simulink model "hyd_hyb_2_int_cont_Final"  (Simulink 8.2)
settings: Solver=ode4  StartTime=0  StopTime=3005  FixedStep=0.01  MaxStep=.4  RelTol=1e-8
InitFcn:
  | const_3_new
values from neighbouring files (symbols this model uses):
  Af = 6.3    [brk_enrg.m]    (also in brk_enrg_1.m)
  BSFC_906_205 = [3.5684 4.3466 5.1668 6.0769 6.988 7.8992 8.8104 9.7336 10.8548 11.9809 13.1112 14.2571 ... (663 elements, 39x17)]    [BSFC_map_906_205.mat]
  Cd = 0.55    [brk_enrg.m]    (also in brk_enrg_1.m)
  den = 1.202    [brk_enrg.m]    (also in brk_enrg_1.m)
  fr = 0.01    [brk_enrg.m]    (also in brk_enrg_1.m)
undefined symbols (not defined in the file or in its folder): clutchRise, down_spd_2, down_spd_3, down_spd_4, down_spd_c, Driving_Cycle, fuel_density, gearshift, I_wheel, Idle_spd_eng_906, M1_hydr, p_v_15, pmax_125, qv_125, Rw, sec_eng_sfc_map, T0, T1, T_max_906, T_min, TC_spd_ratio_max, teta_new_10, torque_convertor, Twait, up_spd_1, up_spd_2, up_spd_3, up_spd_c, v_p_10, v_p_15, v_p_5
libraries: neural x1742, fl_lib x43, nesl_utility x30, sdl_lib x14, simulink x4, simulink_need_slupdate x1
(part 8 of 26)

== system hyd_hyb_2_int_cont_Final/controller1/optimized controller/SOC under 0.5/col_c_d1/net_col_c_d_4_5/Layer 2/LW{2,1} ==
  "ad{2,1}" : Inport  PortDimensions=30
  "IW{2,1}(1,:)'" : Constant  Value=[0.31275731661233508;-0.26985087230257487;0.14779831350765515;0.19073627614307115;0.17869846468081163;-0.4076498321664353;-0.12320323028555259;0.5405778511547239;0.12006388689999251;0.18148367011505864;0.31300573312230928;-0.24996102840664408;-0.26441353396742651;-0.31321873567065162;0.11622017278684436;-0.51269043087096478;0.24925186624599799;-0.51621146910877935;0.33750880398751393;-0.047875273652552772;0.054833649657576623;0.26144850973430128;0.31026665108346058;-0.1108382642077653;-0.23081134064217226;-0.35278496429078965;-0.10237565125670281;-0.21516087744082762;-0.48197610020281068;-0.1586790161425666]
  "IW{2,1}(10,:)'" : Constant  Value=[0.45438550635207459;-0.077905563294043856;0.064273027441706682;0.077966478501816538;0.10808472120474266;0.10911467704478268;-0.16023482762816665;0.18940926466521521;-0.21540812220195904;-0.44805812339676698;0.2672054384669737;-0.26792651540227419;0.20075923623002886;-0.22761094433996942;-0.095380404158750848;-0.084613269916532077;-0.13414255984912157;0.017595198819076098;-0.48675868307727649;0.22485563092185853;0.35538320042057187;0.041419533499156391;0.46339043665268181;0.49721579071234889;0.42207463701328973;-0.18391957358226949;0.24202005592977807;0.47408413991594811;0.52126261687656894;0.11222181265673713]
  "IW{2,1}(11,:)'" : Constant  Value=[0.39457343239192849;0.42458140946112827;-0.27287414777894187;0.067462724870659033;-0.03068429305744165;-0.11770402358430208;-0.37507142879373412;0.34598661664159674;-0.16206818607070139;-0.21370347889050573;0.39446895861921455;-0.14266125325467557;-0.14618395230039505;0.070452872197452027;0.066864440914504428;0.12451211897450633;0.012356818647122547;0.20793588176160319;0.11581661701219066;-0.35814546578829082;0.22455949634467293;0.5468167979497347;-0.55309677720618045;0.18067877568756779;0.00079594352242104113;-0.22857690375549169;-0.53472450281376172;-0.20073202836744419;-0.49233912412032937;0.40992076701468799]
  "IW{2,1}(12,:)'" : Constant  Value=[0.41350579326766701;0.21762640096045338;-0.3097139754237494;-0.2329698564124216;-0.40175947951283236;-0.23814602984300204;-0.51438263530747763;-0.20638550086744714;-0.13770761946706397;0.20930534945632584;0.46082097929918853;0.21897176978274985;-0.27255663625198434;-0.15054029720111464;-0.31656190468089873;0.33873660377538872;-0.018063524886034854;-0.36802746829566002;-0.18497782466494439;-0.19667489988898551;0.15281990588690275;0.27364171079455202;0.33039364278843469;-0.26666673631028642;-0.24425693716621172;0.040179265190829531;0.47861972776555706;0.26460968321609213;0.11706213520914137;-0.31923071600415104]
  "IW{2,1}(13,:)'" : Constant  Value=[-0.38983329555488072;0.10298134054478783;0.21048069589522062;-0.30818809919317486;0.16735156940050316;0.41375380311198673;-0.38987145223320535;-0.35565431169396255;0.22351610936772529;0.25879777713949231;-0.14184756994632572;0.43424468556067913;0.013375203965787376;-0.46400352956380603;-0.27636068442283446;-0.11336907725358317;0.08727021308118893;-0.24264501449480502;0.20756145821823418;0.27346740399021308;-0.42540340708638469;0.19736043169833001;0.44350595567853268;0.19321888665059592;0.37137571007612136;0.34439432357764344;0.27178309423110542;0.39923266521435319;0.13146686845982195;-0.11037819911004416]
  "IW{2,1}(14,:)'" : Constant  Value=[0.21882975012069514;0.1102379619120018;-0.10070141925502289;0.32743984138257093;0.51118972234674531;0.43573443039915827;-0.34375367534563284;0.28860869899214936;-0.027302686712575221;-0.33514454875747118;-0.42624595937362442;0.33248754422370219;-0.21807042688745035;-0.52802984846735068;0.18057289640456653;0.38725540109825934;0.29859268669837774;0.11535303256146118;0.31188442053164722;-0.15890248352815453;-0.061821527024561958;0.11984764110158726;-0.036239661265500982;0.42448419345038174;-0.0040841624827879621;-0.35047521428981115;0.36539965174890987;-0.25151482552180904;0.0043691747446089387;-0.14143232802150388]
  "IW{2,1}(15,:)'" : Constant  Value=[0.40647338431822938;-0.20001708935167542;-0.51281094464128818;0.049782981157163765;-0.17920999529625167;-0.27329699265418117;0.26962913809040551;0.47716366967560603;0.53696090038913025;-0.31255154459434042;-0.029745540476640381;0.1866160633838472;-0.33905178678588266;0.29106755325766553;-0.25821542422978266;-0.24029339121230353;-0.0035892080936714759;0.3194228020317908;0.33761714149176425;0.22697923201352907;-0.077978749273528103;0.050585502149808108;-0.22800546330759139;-0.45058281599612149;0.31595194999031218;0.44829307353340181;-0.27877965028572105;-0.21315229504655123;0.21126039289530585;0.32371351590829367]
  "IW{2,1}(16,:)'" : Constant  Value=[0.068233289188800172;-0.35511628123062366;-0.13456127181794694;-0.11816939495311189;0.35215637018833529;-0.41653092957567556;0.27862712938625833;0.11914056411175804;0.35499529655056261;-0.10061969322539223;0.14120075828841808;0.39501967548068662;0.22237098694536198;0.22753039224917407;-0.1912161648101082;-0.053532058431284404;0.43330060830843981;-0.40135538410096994;0.12027399398626523;-0.29127748746366555;0.22073000400657264;-0.52488192987064708;0.04552877510689797;0.032071827906611852;0.25221796966568777;-0.1246298134168777;0.48349959007046628;0.35217749374902163;-0.43579154396212266;-0.34095381824640847]
  "IW{2,1}(17,:)'" : Constant  Value=[-0.24102258277888214;0.42237910973632548;0.3732244626117559;0.2645155665316376;0.063016448033312911;-0.078422893492473861;0.302057424776629;0.35972686797948694;-0.41651868843111522;0.49899190855904718;-0.46472265979404825;0.005949808915848195;-0.41033968769219381;0.12309139438986795;-0.072517893553310162;0.43612188032541083;-0.336647838886863;0.39085946595790944;-0.32212246749708662;0.014697880621202938;0.12960680979224209;0.10392912461439244;0.074160942133394012;-0.46779281255777821;0.20515478936828335;0.25081088087070574;-0.10698219453587313;-0.21295991077406673;-0.21297824442243884;0.21837942947106137]
  "IW{2,1}(18,:)'" : Constant  Value=[0.059759050225267778;-0.27791706807936212;-0.35008479273333992;0.24878321748016538;0.075872716130115328;-0.0676945295150779;-0.44124907434319061;0.35000632127664316;0.38533241526586348;-0.12361078789315258;-0.082779322297490271;0.15999329415881977;0.042356342806022261;0.29030424704665431;-0.51698206134190861;0.21320259619178908;0.4121019278486926;0.37465473694615287;-0.25132108070492681;-0.11007359828242552;-0.33015522076856618;0.18798249136039627;0.18204609562084603;-0.39665944445609236;-0.41154660905580748;-0.16994986605823159;-0.1692955872746989;-0.084005493488811103;-0.47131807612986337;-0.45578642456255264]
  "IW{2,1}(19,:)'" : Constant  Value=[-0.47886938227031417;0.032469457537400305;-0.25542104742245059;-0.26167394587019804;-0.10238940058752172;0.09748971581301949;0.10986467030249047;-0.22034914411988779;0.26410419478307628;0.19984648446248054;0.10272919448576125;-0.56053811290237565;0.25628511943482707;-0.16813290569704722;0.39759444526884469;0.56965220071070788;0.38494247411175653;0.16530272179566097;-0.048376693521673432;0.21177807584289449;0.37575026242104831;0.30453417835192959;0.31565094074247002;0.1676691940210048;-0.033954839293835484;-0.28130350691137318;0.18751282661063398;0.29791372323587106;0.48208294523816858;-0.24731324303734542]
  "IW{2,1}(2,:)'" : Constant  Value=[0.16485594905702061;0.41958460563899208;-0.087556982214553172;0.099659077192037468;-0.34322740388705358;-0.3233151486552453;-0.41887378222277061;0.046432114993733058;-0.04898360854476292;0.16153529016460713;0.28844117833541272;-0.29776282115080782;0.25010799495268621;-0.50504804649059543;0.23860604320730203;-0.34818567250330251;0.33046575769726333;-0.46398401002715511;0.09588243880572192;-0.28059551643412539;-0.25844161306811819;0.19187556916319429;-0.22646588144013996;-0.12620457794262144;-0.38984869350840334;0.50675143299656611;0.11659348313501641;0.11930517585189776;-0.38665943551255716;0.15213966711994284]
  "IW{2,1}(20,:)'" : Constant  Value=[-0.50349152720019708;-0.15010554830208991;0.04823860371701947;0.21563733179354533;0.17870399256241923;0.36223693131943974;-0.17259449670673224;-0.15585032550862551;-0.30294761986714053;0.40528052511574736;0.062050664964907888;-0.029356423222545683;-0.29477014410269187;0.058391152070021719;-0.47589128512679713;0.53116788114847968;0.1868250849425496;0.040929221667824277;0.38990550796746748;0.24300137252896023;0.10615772766965213;-0.12223235512275682;-0.38620447778361577;0.10284616000000632;-0.53191757250801641;0.060123296195749305;0.42009066845053133;-0.081139615013162442;0.28050737924076169;-0.39610717394304934]
  "IW{2,1}(21,:)'" : Constant  Value=[0.27654849170357604;0.44000998144944226;0.34978032343014748;0.16287626128560476;-0.31106448364869971;0.2712986975363621;0.17477184643602001;-0.040994417241635855;0.040756820710299513;-0.32217945823032945;0.033526998625739449;0.28083486484077141;0.07527788850813795;0.031141752002320815;-0.13842179269689114;-0.44467088615542294;0.16343581497338305;-0.25175895155410183;0.37296608238294682;-0.26225689114314404;0.036532039732935541;0.57172449283776772;0.11563544110226888;-0.41021444626899761;0.24900514830006129;0.29631891929786808;0.42548416020169089;0.42501941439136554;0.66763009748879998;0.03027871495198993]
  "IW{2,1}(22,:)'" : Constant  Value=[0.38175362027160537;-0.2376980384911867;-0.30063107682478601;-0.33881306444168069;0.17849746917857029;-0.34964626211640071;0.47826477896920283;-0.45640710628278391;-0.27942561203021932;0.40006277245588362;0.12139177090538589;0.23428665944684432;0.47448510322777709;0.0048315672861399079;-0.062689816480599722;0.060400310154686547;-0.20714240476303258;-0.42676738802132902;0.33105522009343091;0.063936510689872036;-0.17953036149592752;-0.27004097229269541;0.45556337239058609;-0.18429429231486444;-0.34003366383251599;0.24510978349593487;-0.1936015912949566;-0.21466624872492407;0.14985155313151818;0.054107134676608881]
  "IW{2,1}(23,:)'" : Constant  Value=[0.19208517656566945;-0.23756553933116847;-0.40298748221062619;0.315881501215938;0.33300767958814698;0.054607137245660312;0.070510839064599679;0.25843945839112381;-0.47818192403809279;-0.22121986735846599;-0.42796937877860231;0.28019957286856068;-0.42271140569854398;0.24074409826905843;-0.2382457659414558;0.31288621521010146;-0.10634533622057268;-0.42795872100881838;0.33242045568973272;0.27235300570836396;0.4452188850608414;0.25216641636573384;0.42859453638665451;0.042237698775830494;-0.010407092153751055;0.27847694370500309;0.037030252368509826;0.24700161997172382;-0.2740168070269105;-0.051812001981064143]
  "IW{2,1}(24,:)'" : Constant  Value=[-0.25041942582150839;-0.4783743097785057;0.33758877202355092;-0.35771582757284054;-0.069784976792996542;-0.18183718522479581;-0.29647307869149248;-0.01258022132651891;-0.38608590463206277;-0.17128957156155242;0.28378323654610887;-0.1232662979796499;-0.034840090696733474;-0.21583788403895016;-0.35856711536397545;0.27291622414266103;-0.48944471164387804;-0.17030385013592783;-0.31970851699994202;0.17182723354569193;-0.050945541622091077;-0.2331708593756367;-0.0011402081132685206;0.40596696938193017;0.30363557399044233;-0.2771351555329063;0.35320261019636923;-0.27312545966154628;0.50923636237666603;0.22586347700180542]
  "IW{2,1}(25,:)'" : Constant  Value=[0.32349444512379921;0.074648383376890656;0.18340658341772714;0.43907131187832443;0.24465430553770609;0.23034266690144972;0.47224773188761382;-0.039851790753156688;-0.28799592424079162;0.46792175397215163;-0.052747978840832654;0.18850645864976925;-0.23554460115113637;-0.19364311776843482;0.35316221950874893;0.44064660342413975;0.18917215303582707;-0.12420884828585119;0.40538631794931379;0.22819341411136568;0.059594500015362512;0.28343720639866427;-0.45140839586712117;0.1478703357973816;0.30076697778334688;0.15221057482232195;0.035957199643899887;-0.17933932303548003;-0.41443602301923138;0.42878258387315454]
  "IW{2,1}(26,:)'" : Constant  Value=[0.36591493875311448;0.42528293161766884;-0.30435369071635565;0.14276477985755814;-0.04495075026453995;0.19809379202781327;0.51087121120446755;0.21486333322079815;-0.34059850815575499;0.084745163469986964;-0.30926516084598771;-0.07546102676902644;-0.12460229619037608;0.18508313015789429;0.12897811993832092;-0.22442795556708969;0.019023619473468013;0.34747781394647176;-0.37296250313818691;-0.028844860117835443;0.30287166816632488;-0.18991160260759973;-0.41896864492380009;0.0032567424690979675;-0.28457586214599073;0.21844863504622525;0.18315065831218991;-0.46689768004420179;0.65930160457142706;-0.50391368734202047]
  "IW{2,1}(27,:)'" : Constant  Value=[-0.45165726459295841;0.18685298448002466;-0.0090335448745681585;-0.52954877861384042;-0.14477143023223485;0.045597100123252285;-0.29536340634700303;-0.19327933685493373;0.24862380838491852;0.19703321893290365;0.5107467939404432;-0.16533346090025589;-0.26226009715655274;-0.15632117807422943;-0.063571615898426373;0.55995701861756586;-0.53001173127896606;-0.19441677800206064;0.076824338048925925;-0.11179108588524951;-0.14135238157903199;0.39349867681877754;0.023404631751319238;0.37216463490856705;0.53159287863188354;-0.282683317094924;-0.1273085783656768;-0.11809939138651696;0.062648977706862341;0.01948150734503756]
  "IW{2,1}(28,:)'" : Constant  Value=[-0.58060952775684338;-0.22557606247832096;0.52097869943267794;-0.19586163071942558;0.0062674764494588262;-0.066850020962621756;0.20177734453309737;-0.27847284591627308;0.33847362494561467;0.35269036115819041;0.39821372354421114;-0.075296913241820349;-0.2104646699645738;0.44653380119651459;-0.18745831379084438;-0.60540044413148164;-0.082560268753580454;0.010533100539155408;0.093177597410024335;0.029253479090595141;-0.035674987634033255;-0.20045674250673423;-0.30562918019644403;-0.24631105348707522;0.045490458801701883;0.059752260576021003;0.55791046780256159;0.19353601707602536;0.28902863117259614;0.066799928097732178]
  "IW{2,1}(29,:)'" : Constant  Value=[0.200626701170141;0.11341200725191816;0.25400945898747868;-0.29711962816610615;-0.25863315355850092;0.35744982028032246;-0.5080920038212503;0.58181325676261442;-0.097398879041334083;-0.12638833145718376;-0.10014932495998892;-0.28239825293861465;-0.2339851544517525;0.14485834314410745;-0.25498351212539166;0.045186437575171177;0.59327181045491273;-0.60524360933909438;0.25456298981177006;-0.18584367266637661;0.12303436253633954;-0.042955730385764286;0.42151102793510242;-0.23533227271142015;0.10481495152121964;0.0024264444668975877;-0.032072789036909792;0.28820697053753419;-0.24353411968483479;0.17434993503616078]
  "IW{2,1}(3,:)'" : Constant  Value=[0.3459096676297157;-0.11796751712458815;0.46227598264851438;0.14263353014580396;0.34214145196121382;0.067536028640059004;-0.4308090682770192;-0.26595770030532756;-0.40464381327048471;-0.41297978470556329;-0.083143061155957307;-0.2213102003231478;0.28674899904423712;-0.25566004614728211;-0.2637262681895613;-0.19672965570919757;0.42630776831842748;-0.23603035795505956;0.18479113555339288;0.13330554053305646;-0.44289673634078358;-0.22028406519497015;-0.071392960615195372;-0.2619638898003428;-0.27848765975481171;0.31573980431370213;-0.29837469379576242;-0.4458157730139885;0.064506187512735597;-0.11504288424397838]
  "IW{2,1}(30,:)'" : Constant  Value=[0.15190325397518098;-0.34216215066573985;-0.39814751560646894;-0.42943267994355339;-0.21875047919699234;-0.21287914075563277;-0.27073826951352659;-0.42295417300718602;0.32460992703246305;-0.43774963439841746;0.061558139773068475;-0.019684675811075684;0.42020559123125811;-0.39776452768660175;-0.5234335532592449;-0.16168817301124472;0.14003142322982184;0.10628363934677905;-0.086823016807298495;-0.046194531903006285;-0.033725503218865346;-0.41006731661327178;-0.34684589361002549;0.082045516770265753;-0.28831677388251697;0.38628769766659182;0.28636646919507447;-0.14510905709409513;0.29510810475862387;-0.21942176632829943]
  "IW{2,1}(31,:)'" : Constant  Value=[-0.39196147587405461;-0.30484384520281688;0.32339020886236586;-0.24533783720737751;-0.28243060314126101;0.35853256400686745;-0.096180248562639889;-0.3031052656978025;-0.46296078164800541;0.017110740095564039;0.24319533946695593;-0.14594960536939233;-0.46901714224314928;-0.42991556788729024;-0.24347837627827257;0.49572366809363572;-0.3711206454426727;-0.078473534413682378;-0.18768615924301743;-0.19917658263020099;-0.36562820167011711;-0.060476596214022328;0.22652353361504782;0.082677122740594522;-0.27809312170130696;0.14116400393821171;-0.37520933679946206;0.20713872373871514;-0.12846495534626934;-0.26230599104356522]
  "IW{2,1}(32,:)'" : Constant  Value=[-0.27915563919657271;0.0031543366869891116;-0.074356213945820829;0.60541914834384591;0.21906474630133854;0.053542864961575495;-0.41393610408740883;0.049831763478782272;-0.59172997102716274;-0.21372816909418876;-0.47611585362483089;0.024910784918673722;-0.6694666312496329;0.082460309831931727;-0.17015304403916198;-0.070164320290546353;0.047563633318013374;-0.34828596499173975;0.039615165090038554;-0.22770922258295684;0.12685346317662261;0.5812308928526484;-0.26687408138421853;-0.10678767449453988;-0.30871960935658288;0.080909724361547933;-0.065676115606442972;-0.17599364507922607;-0.15345393026672444;-0.13957577397509063]
  "IW{2,1}(33,:)'" : Constant  Value=[-0.14241530488200782;-0.42802886140837171;0.22382159633187695;-0.23395685062514587;-0.43289738365933766;-0.33881337748403562;-0.2807740627158769;-0.18296096952563212;0.33633354136552684;-0.095685317058735384;-0.36551851743406943;0.45398299496209066;-0.14601089686704719;0.39142342911155814;-0.27831665329158656;0.21541539538043869;-0.36029628835130523;-0.43108890247934833;0.18302081726576166;0.084393873101736697;0.3259336830432813;0.41589742614527048;0.26087955589125039;-0.21282332443442339;-0.24557835715225795;-0.027545930655320287;-0.31727289221876193;-0.26420356879217649;0.15847775495593014;0.18198182070612359]
  "IW{2,1}(34,:)'" : Constant  Value=[-0.1080813176840188;0.031877423816805729;0.43003917155021437;-0.19446938568529362;-0.4638454953879948;-0.23757477543062727;0.032996428279117494;-0.23966793739279438;0.38410933344413728;0.15240169782027815;-0.42872348965582635;-0.020835572776745432;0.17700773516150659;0.48990883523550122;0.37097995759145441;-0.30512589395578371;-0.44608773131815127;0.32579486658577667;0.39636767324860256;0.1807027895135021;0.23749883582488848;-0.24971507549780828;-0.36185798007397568;0.48185320598392634;-0.11417150403539712;-0.072485959616476234;-0.18977680507334568;0.0087344840836283879;0.19591929810703587;-0.1611155049720481]
  "IW{2,1}(35,:)'" : Constant  Value=[0.28637756011481041;-0.01883311693596772;0.4032250294391555;-0.1620436547326822;-0.51840640598156196;-0.43210195154936415;0.29892194265780975;-0.010068380822181065;-0.032801409050717385;-0.094579120494082611;0.084606294379177452;-0.3250088029757065;-0.17473214707481291;-0.21568918324783523;-0.43287752741456603;0.46279201783067719;-0.002324495961844919;0.13076008214567994;-0.28600464486555599;-0.23721237794517117;0.11391355774762742;-0.41839662000656508;-0.51413807719874494;0.18575832928932814;0.18961472877535523;-0.089024071548704786;0.48390714533162726;0.11636984161140511;0.34653536649007477;-0.17927531322005694]
  "IW{2,1}(36,:)'" : Constant  Value=[-0.36210314109763053;0.14584188290398084;-0.35438442449050594;0.32315450009904317;0.18434784726834644;0.38493084551990348;-0.096535485247892447;-0.18658324859701786;-0.046754406456686326;0.51074777088191625;0.31481372129285495;0.37681683213926354;-0.32036486099036615;0.017548820888744331;0.4009661821533998;0.098167186415540009;0.23451840361056001;0.39521897549836915;0.041940753905107306;0.28840714311974119;0.092321041979203114;0.25009242632983703;0.25803285198791565;-0.46282207162139155;0.40890961979162882;0.021747727427568642;-0.49511963345440418;-0.20447453933880586;0.047925656474884122;0.14473490628736754]
  "IW{2,1}(37,:)'" : Constant  Value=[0.30895980101971848;0.2205995057081224;0.014215062392222162;-0.35743246531383871;0.078114912171393075;-0.3716774172840871;0.18963429706101939;0.094014671548542858;-0.30483996969855698;0.27231359653796966;-0.21558939931622154;0.20737577142209412;-0.33794212840815074;-0.16422042277311097;-0.432186262416135;0.44347392277162362;-0.28376178074835973;0.092808417192934811;0.23982683239387254;-0.057619954301717249;-0.1502789954807599;-0.50024378241445777;-0.055461327531646114;0.15889498771577498;-0.49528223882524575;0.54437730654311189;-0.33165473512905069;-0.26995389111620571;0.20230457029389584;0.083413067871219063]
  "IW{2,1}(38,:)'" : Constant  Value=[0.31376155073349921;0.38735585542746392;0.11982352708142101;-0.44485010346037318;0.2538529549617653;0.12326898087066515;0.19627230873225621;-0.12292507361069381;0.44732019656864452;0.21381392787092793;-0.10540473725430266;0.046547911838308614;-0.26005530486766804;-0.092360969592290634;-0.35643113638449714;-0.30793831072341116;0.42038732950729013;0.40916985478650209;0.22768604915972937;-0.34754216788287967;-0.098971341532745671;0.39545233206496044;-0.41400939765243283;-0.1522799472065576;0.16999513541993228;-0.30420322783241793;0.094578321305834573;-0.26622295727616196;0.36998948162013501;0.37491396323200438]
  "IW{2,1}(39,:)'" : Constant  Value=[-0.0020064593389496049;0.42463890271185478;-0.084869246006223503;0.13312921673087996;-0.35561987529069944;-0.1631643953339536;-0.10922694340892829;-0.06765434448875729;0.037078984117479584;0.039871739277738717;-0.14593915974365232;0.43656333330665248;0.26261588008845604;-0.39756482931894077;-0.41914777810315396;-0.41721262966073996;0.49922918699183166;0.097945865589809181;-0.25934109090236468;-0.40641397794973788;-0.49046253407477991;0.23959196411459993;0.022923979689467112;0.26567613392988421;0.34004535213417464;-0.48963607367670614;0.17405455279805812;-0.11888857301090927;-0.29101122979555866;0.022759802472809038]
  "IW{2,1}(4,:)'" : Constant  Value=[0.24884602764519553;0.011662817403598679;0.30004204405401175;-0.30213030285491976;-0.37240048328027758;-0.063612854437861036;0.16885727465472147;-0.19920232018388431;-0.4327371635069609;0.3281653159173003;0.24440163725476829;-0.40961038191572063;-0.32071974797282893;-0.22574883055005474;-0.40258802248002623;-0.38044163556309479;0.28940501837107774;-0.36724248494394268;-0.36539679359632593;-0.13576889895403829;0.096013382386674506;0.15767164369658879;-0.35887994422675973;-0.26090216467487937;-0.35986426731161514;-0.44831164855973205;0.19102962307798715;0.12934044546397921;-0.090685632702068183;0.24438127240792426]
  "IW{2,1}(40,:)'" : Constant  Value=[0.47231305767361814;-0.4435329241076687;-0.29471890313503751;-0.29445184768907751;-0.1288902727338922;0.42178628341168645;-0.17367845551935812;-0.011520243983458654;0.063013213396622705;-0.30807790612722352;-0.10467980927399435;-0.34730373262865949;0.032801004445701464;0.0012963986235965555;-0.13888340651489126;0.32696783648073474;-0.31576075422582089;0.21365430733274085;-0.4134871672491357;0.31745202000616701;-0.12498690934146456;-0.2947331210328587;0.45129695059181368;0.43023017404594532;-0.35936441760492538;-0.44554958440007569;0.17420016060189544;0.12202951393332437;0.20479294535271642;-0.077817926858881906]
  "IW{2,1}(5,:)'" : Constant  Value=[-0.062901709304139783;0.32341137965665484;0.050527689980782754;-0.16487151299127989;-0.045815962388067497;0.50511421457259975;-0.18013089336815724;0.061715070505560118;0.28235840385390576;-0.39856132729554111;0.0023061732376174794;-0.23449982892962193;0.38952129699583593;-0.011440048982628416;0.40942338391488875;-0.39827020000003011;0.023525814677469354;-0.2186305674801248;0.52230031676125732;0.41492987436367007;-0.42941454695237141;-0.15360167182139192;0.27769917090917323;-0.4266750314682079;0.35265544711904667;-0.048369340187480195;0.045767014999578512;-0.019588517841915076;-0.36491651405831882;0.30534704709780569]
  "IW{2,1}(6,:)'" : Constant  Value=[0.14649388353113663;-0.22457556384651209;0.41114328992622839;-0.40380519063788617;0.46424038683218355;-0.34306115074364552;-0.40919766016808684;-0.048929718916915249;-0.41471276760485898;-0.28448059873982734;0.42312029090984776;-0.10463115287581726;-0.13722175612637078;0.11679976409816603;-0.22948999051804081;0.064769205503860949;-0.24089725871610537;-0.23693643690607052;-0.29211385277033741;0.073667883044920585;-0.46627822849915135;-0.25574129709186616;-0.103535859979867;-0.2874562200965296;-0.27565493511549399;-0.20832958498408963;0.47443704695435779;0.36303048561885215;0.14695330736401896;0.046696723471653406]
  "IW{2,1}(7,:)'" : Constant  Value=[-0.28369330135027643;-0.28247025426586919;-0.29327005551695901;0.33716826498283092;0.27667110389940391;-0.10852914106983955;-0.39616325954735659;0.31312232949019919;0.16069907041519635;-0.21407336364033694;0.29314107740163425;-0.082119025675407215;0.27377487239493759;0.010940682067417256;0.198272649173522;0.40906242406446958;-0.15188119293446137;-0.35309753913457093;-0.38016952468941689;0.40029450234037023;0.12759173703826107;-0.33040256725861405;-0.2703842078354089;0.33484452581795426;-0.35398015747574452;-0.010795853196711971;0.34312537372447;-0.053240154935927826;0.34412665912292595;0.37251434655521104]
  "IW{2,1}(8,:)'" : Constant  Value=[-0.20923284873373496;0.24554235823081641;0.27407254142511789;-0.08214097632887632;-0.21240424957991907;-0.32026505432150049;0.4388254076141479;-5.1044985481562587e-005;-0.39064340534512793;-0.4149544427086127;-0.39537804980330282;-0.34694923824881235;0.19431640822985691;-0.36321375493294389;0.14098683810873255;0.34412516279956412;-0.023064918854102036;0.20078487216987131;-0.18711800366799441;-0.29535806023912431;0.068030782603948875;-0.265067842092996;-0.12145593370504683;-0.47512489122608942;0.38230144593675691;-0.075320862525029911;-0.33328505959559945;0.39182886243929138;-0.22974155825193956;-0.44096692163984375]
  "IW{2,1}(9,:)'" : Constant  Value=[-0.38273875807747837;-0.53038263554913556;0.07663390557537525;0.3517524726482894;-0.36880503061111952;0.26994520408226053;0.1154625386840097;0.042636040009437715;0.44297428848937392;-0.38061478854327563;-0.47190766217819219;0.25615755069572643;0.3584017357215783;0.067414172681270007;-0.20091641281789024;0.213782292714123;0.077085749553810076;-0.1050348327444577;-0.28870725365274741;0.0038040324511218154;0.136175748417838;-0.34565268641657898;-0.33113569859445707;0.050391119456636949;-0.32682675250849214;-0.20582404721348957;0.36911869262913682;0.070626392320243411;-0.027000597528334495;0.46817855347483345]
  Mux : Mux  Inputs=40
  dotprod{1..40} (40 alike) : neural/Weight Functions/dotprod
  "lz{2,1}" : Outport
  wires:
  Mux/1 -> "lz{2,1}"/1
  dotprod40/1 -> Mux/40
  "IW{2,1}(40,:)'"/1 -> dotprod40/1
  dotprod39/1 -> Mux/39
  "IW{2,1}(39,:)'"/1 -> dotprod39/1
  dotprod38/1 -> Mux/38
  "IW{2,1}(38,:)'"/1 -> dotprod38/1
  dotprod37/1 -> Mux/37
  "IW{2,1}(37,:)'"/1 -> dotprod37/1
  dotprod36/1 -> Mux/36
  "IW{2,1}(36,:)'"/1 -> dotprod36/1
  dotprod35/1 -> Mux/35
  "IW{2,1}(35,:)'"/1 -> dotprod35/1
  dotprod34/1 -> Mux/34
  "IW{2,1}(34,:)'"/1 -> dotprod34/1
  dotprod33/1 -> Mux/33
  "IW{2,1}(33,:)'"/1 -> dotprod33/1
  dotprod32/1 -> Mux/32
  "IW{2,1}(32,:)'"/1 -> dotprod32/1
  dotprod31/1 -> Mux/31
  "IW{2,1}(31,:)'"/1 -> dotprod31/1
  dotprod30/1 -> Mux/30
  "IW{2,1}(30,:)'"/1 -> dotprod30/1
  dotprod29/1 -> Mux/29
  "IW{2,1}(29,:)'"/1 -> dotprod29/1
  dotprod28/1 -> Mux/28
  "IW{2,1}(28,:)'"/1 -> dotprod28/1
  dotprod27/1 -> Mux/27
  "IW{2,1}(27,:)'"/1 -> dotprod27/1
  dotprod26/1 -> Mux/26
  "IW{2,1}(26,:)'"/1 -> dotprod26/1
  dotprod25/1 -> Mux/25
  "IW{2,1}(25,:)'"/1 -> dotprod25/1
  dotprod24/1 -> Mux/24
  "IW{2,1}(24,:)'"/1 -> dotprod24/1
  dotprod23/1 -> Mux/23
  "IW{2,1}(23,:)'"/1 -> dotprod23/1
  dotprod22/1 -> Mux/22
  "IW{2,1}(22,:)'"/1 -> dotprod22/1
  dotprod21/1 -> Mux/21
  "IW{2,1}(21,:)'"/1 -> dotprod21/1
  dotprod20/1 -> Mux/20
  "IW{2,1}(20,:)'"/1 -> dotprod20/1
  dotprod19/1 -> Mux/19
  "IW{2,1}(19,:)'"/1 -> dotprod19/1
  dotprod18/1 -> Mux/18
  "IW{2,1}(18,:)'"/1 -> dotprod18/1
  dotprod17/1 -> Mux/17
  "IW{2,1}(17,:)'"/1 -> dotprod17/1
  dotprod16/1 -> Mux/16
  "IW{2,1}(16,:)'"/1 -> dotprod16/1
  dotprod15/1 -> Mux/15
  "IW{2,1}(15,:)'"/1 -> dotprod15/1
  dotprod14/1 -> Mux/14
  "IW{2,1}(14,:)'"/1 -> dotprod14/1
  dotprod13/1 -> Mux/13
  "IW{2,1}(13,:)'"/1 -> dotprod13/1
  dotprod12/1 -> Mux/12
  "IW{2,1}(12,:)'"/1 -> dotprod12/1
  dotprod11/1 -> Mux/11
  "IW{2,1}(11,:)'"/1 -> dotprod11/1
  dotprod10/1 -> Mux/10
  "IW{2,1}(10,:)'"/1 -> dotprod10/1
  dotprod9/1 -> Mux/9
  "IW{2,1}(9,:)'"/1 -> dotprod9/1
  dotprod8/1 -> Mux/8
  "IW{2,1}(8,:)'"/1 -> dotprod8/1
  dotprod7/1 -> Mux/7
  "IW{2,1}(7,:)'"/1 -> dotprod7/1
  dotprod6/1 -> Mux/6
  "IW{2,1}(6,:)'"/1 -> dotprod6/1
  dotprod5/1 -> Mux/5
  "IW{2,1}(5,:)'"/1 -> dotprod5/1
  dotprod4/1 -> Mux/4
  "IW{2,1}(4,:)'"/1 -> dotprod4/1
  dotprod3/1 -> Mux/3
  "IW{2,1}(3,:)'"/1 -> dotprod3/1
  dotprod2/1 -> Mux/2
  "IW{2,1}(2,:)'"/1 -> dotprod2/1
  dotprod1/1 -> Mux/1
  "ad{2,1}"/1 -> dotprod40/2, dotprod39/2, dotprod38/2, dotprod37/2, dotprod36/2, dotprod35/2, dotprod34/2, dotprod33/2, dotprod32/2, dotprod31/2, dotprod30/2, dotprod29/2, dotprod28/2, dotprod27/2, dotprod26/2, dotprod25/2, dotprod24/2, dotprod23/2, dotprod22/2, dotprod21/2, dotprod20/2, dotprod19/2, dotprod18/2, dotprod17/2, dotprod16/2, dotprod15/2, dotprod14/2, dotprod13/2, dotprod12/2, dotprod11/2, dotprod10/2, dotprod9/2, dotprod8/2, dotprod7/2, dotprod6/2, dotprod5/2, dotprod4/2, dotprod3/2, dotprod2/2, dotprod1/2
  "IW{2,1}(1,:)'"/1 -> dotprod1/1

== system hyd_hyb_2_int_cont_Final/controller1/optimized controller/SOC under 0.5/col_c_d1/net_col_c_d_4_5/Layer 3/Delays 1 ==
  "p{3}" : Inport  PortDimensions=40
  mux : Mux  Inputs=1
  "pd{3,2}" : Outport
  wires:
  mux/1 -> "pd{3,2}"/1
  "p{3}"/1 -> mux/1

== system hyd_hyb_2_int_cont_Final/controller1/optimized controller/SOC under 0.5/col_c_d1/net_col_c_d_4_5/Layer 3/LW{3,2} ==
  "ad{3,2}" : Inport  PortDimensions=40
  "IW{3,2}(1,:)'" : Constant  Value=[-0.43141211792559142;-0.11888165414139513;-0.22701302193417633;0.14315500955996635;-0.11268052842329422;-0.66755337377971913;-0.90374763549360537;-0.76985267606758923;-0.62023649272464287;0.19138878884193214;0.99640825481026107;0.30069820196235497;-0.90113832366665458;-0.69317441551269632;1.0524663804640109;0.40315249365778993;0.8257560441646864;-0.43196133618180077;-0.62424800501186883;0.74264769849740953;0.99995606798411707;-0.13032239355778821;0.71476098102029351;0.92404578703104456;0.075939871013732146;0.94468909976236903;0.19330991737906994;0.47787649449252922;0.89436963345916265;-0.79706254287066325;-0.01014931738240097;0.58899206441818175;0.98972787944860419;-0.19553007982111831;-0.10078290415230909;-0.26312481872565424;-0.80903105213119841;0.38143504933278732;-0.098828531512075504;0.27196209686502049]
  Mux : Mux  Inputs=1
  dotprod1 : neural/Weight Functions/dotprod
  "lz{3,2}" : Outport
  wires:
  Mux/1 -> "lz{3,2}"/1
  dotprod1/1 -> Mux/1
  "ad{3,2}"/1 -> dotprod1/2
  "IW{3,2}(1,:)'"/1 -> dotprod1/1

== system hyd_hyb_2_int_cont_Final/controller1/optimized controller/SOC under 0.5/col_e_f/net_col_e_f_2_4/Layer 1/Delays 1 ==
  "p{1}" : Inport  PortDimensions=2
  mux : Mux  Inputs=1
  "pd{1,1}" : Outport
  wires:
  "p{1}"/1 -> mux/1
  mux/1 -> "pd{1,1}"/1

== system hyd_hyb_2_int_cont_Final/controller1/optimized controller/SOC under 0.5/col_e_f/net_col_e_f_2_4/Layer 1/IW{1,1} ==
  "pd{1,1}" : Inport  PortDimensions=2
  "IW{1,1}(1,:)'" : Constant  Value=[-2.6649767493760956;-1.5305742272763116]
  "IW{1,1}(2,:)'" : Constant  Value=[-2.686906454238835;-1.6060629338452583]
  "IW{1,1}(3,:)'" : Constant  Value=[-0.67354865862732705;-2.9466944922974565]
  "IW{1,1}(4,:)'" : Constant  Value=[-3.1130331362360333;0.74929650760552868]
  "IW{1,1}(5,:)'" : Constant  Value=[-2.2443406365938872;2.1144076594502548]
  Mux : Mux  Inputs=5
  dotprod{1..5} (5 alike) : neural/Weight Functions/dotprod
  "iz{1,1}" : Outport
  wires:
  "IW{1,1}(1,:)'"/1 -> dotprod1/1
  "pd{1,1}"/1 -> dotprod1/2, dotprod2/2, dotprod3/2, dotprod4/2, dotprod5/2
  dotprod1/1 -> Mux/1
  "IW{1,1}(2,:)'"/1 -> dotprod2/1
  dotprod2/1 -> Mux/2
  "IW{1,1}(3,:)'"/1 -> dotprod3/1
  dotprod3/1 -> Mux/3
  "IW{1,1}(4,:)'"/1 -> dotprod4/1
  dotprod4/1 -> Mux/4
  "IW{1,1}(5,:)'"/1 -> dotprod5/1
  dotprod5/1 -> Mux/5
  Mux/1 -> "iz{1,1}"/1

== system hyd_hyb_2_int_cont_Final/controller1/optimized controller/SOC under 0.5/col_e_f/net_col_e_f_2_4/Layer 2/Delays 1 ==
  "p{2}" : Inport  PortDimensions=5
  mux : Mux  Inputs=1
  "pd{2,1}" : Outport
  wires:
  "p{2}"/1 -> mux/1
  mux/1 -> "pd{2,1}"/1

== system hyd_hyb_2_int_cont_Final/controller1/optimized controller/SOC under 0.5/col_e_f/net_col_e_f_2_4/Layer 2/LW{2,1} ==
  "ad{2,1}" : Inport  PortDimensions=5
  "IW{2,1}(1,:)'" : Constant  Value=[0.56460072480523527;-0.27728941529256795;-1.3042050610072675;1.6908339776204973;-0.19900178338510283]
  "IW{2,1}(10,:)'" : Constant  Value=[-0.13270560297571152;1.3554438954941257;0.6115334718676394;-0.64694828900610291;-1.7809391518893904]
  "IW{2,1}(2,:)'" : Constant  Value=[0.10351622638523233;-0.67307222164478875;-1.339714602609521;1.4194941208869205;-0.58174693113686593]
  "IW{2,1}(3,:)'" : Constant  Value=[-1.1298116217383789;-0.97253046033897872;1.2380780562762508;0.44857797804197275;0.98496368265779355]
  "IW{2,1}(4,:)'" : Constant  Value=[0.9571096593892815;-1.414092713071226;-1.2160568547820836;0.31489306555233132;-0.78400492918201437]
  "IW{2,1}(5,:)'" : Constant  Value=[0.2576491260568628;-1.6698639898425696;-1.1690213673727601;0.73581081089882483;0.18447965955190423]
  "IW{2,1}(6,:)'" : Constant  Value=[-1.1142645189890759;-0.93809254894978766;-1.2125692713736391;-0.56637477498120159;-0.98110019103546331]
  "IW{2,1}(7,:)'" : Constant  Value=[-1.1961693981497983;-0.45846373796771644;0.41618641925179262;-0.17199875977727455;-1.7386853209643456]
  "IW{2,1}(8,:)'" : Constant  Value=[-0.58973681219214769;-0.19462836353215293;-0.45483379377550731;0.47226993866583578;2.0255431960466965]
  "IW{2,1}(9,:)'" : Constant  Value=[1.0371946551130358;-1.1601642525597882;0.99734768943716734;0.97772652549464856;-0.74493870033863852]
  Mux : Mux  Inputs=10
  dotprod{1..10} (10 alike) : neural/Weight Functions/dotprod
  "lz{2,1}" : Outport
  wires:
  "IW{2,1}(1,:)'"/1 -> dotprod1/1
  "ad{2,1}"/1 -> dotprod1/2, dotprod2/2, dotprod3/2, dotprod4/2, dotprod5/2, dotprod6/2, dotprod7/2, dotprod8/2, dotprod9/2, dotprod10/2
  dotprod1/1 -> Mux/1
  "IW{2,1}(2,:)'"/1 -> dotprod2/1
  dotprod2/1 -> Mux/2
  "IW{2,1}(3,:)'"/1 -> dotprod3/1
  dotprod3/1 -> Mux/3
  "IW{2,1}(4,:)'"/1 -> dotprod4/1
  dotprod4/1 -> Mux/4
  "IW{2,1}(5,:)'"/1 -> dotprod5/1
  dotprod5/1 -> Mux/5
  "IW{2,1}(6,:)'"/1 -> dotprod6/1
  dotprod6/1 -> Mux/6
  "IW{2,1}(7,:)'"/1 -> dotprod7/1
  dotprod7/1 -> Mux/7
  "IW{2,1}(8,:)'"/1 -> dotprod8/1
  dotprod8/1 -> Mux/8
  "IW{2,1}(9,:)'"/1 -> dotprod9/1
  dotprod9/1 -> Mux/9
  "IW{2,1}(10,:)'"/1 -> dotprod10/1
  dotprod10/1 -> Mux/10
  Mux/1 -> "lz{2,1}"/1

== system hyd_hyb_2_int_cont_Final/controller1/optimized controller/SOC under 0.5/col_e_f/net_col_e_f_2_4/Layer 3/Delays 1 ==
  "p{3}" : Inport  PortDimensions=10
  mux : Mux  Inputs=1
  "pd{3,2}" : Outport
  wires:
  "p{3}"/1 -> mux/1
  mux/1 -> "pd{3,2}"/1

== system hyd_hyb_2_int_cont_Final/controller1/optimized controller/SOC under 0.5/col_e_f/net_col_e_f_2_4/Layer 3/LW{3,2} ==
  "ad{3,2}" : Inport  PortDimensions=10
  "IW{3,2}(1,:)'" : Constant  Value=[-0.60647383905036167;-1.3167916347948412;-0.01345915035995135;0.62162325620354042;-0.18455126173871639;-0.079939564037496691;0.17647220789393392;0.58945842219999534;0.078231552949098629;-0.389216405357934]
  Mux : Mux  Inputs=1
  dotprod1 : neural/Weight Functions/dotprod
  "lz{3,2}" : Outport
  wires:
  "IW{3,2}(1,:)'"/1 -> dotprod1/1
  "ad{3,2}"/1 -> dotprod1/2
  dotprod1/1 -> Mux/1
  Mux/1 -> "lz{3,2}"/1

== system hyd_hyb_2_int_cont_Final/controller1/optimized controller/SOC under 0.5/col_e_f/net_col_e_f_4_5/Layer 1/Delays 1 ==
  "p{1}" : Inport  PortDimensions=2
  mux : Mux  Inputs=1
  "pd{1,1}" : Outport
  wires:
  "p{1}"/1 -> mux/1
  mux/1 -> "pd{1,1}"/1

== system hyd_hyb_2_int_cont_Final/controller1/optimized controller/SOC under 0.5/col_e_f/net_col_e_f_4_5/Layer 1/IW{1,1} ==
  "pd{1,1}" : Inport  PortDimensions=2
  "IW{1,1}(1,:)'" : Constant  Value=[-0.53810010237953376;-6.2269929058788556]
  "IW{1,1}(10,:)'" : Constant  Value=[-5.6641478561689178;-2.6826445370991689]
  "IW{1,1}(11,:)'" : Constant  Value=[3.9208019826789777;-4.9204554738968254]
  "IW{1,1}(12,:)'" : Constant  Value=[-1.7774068275586459;6.088189001348475]
  "IW{1,1}(13,:)'" : Constant  Value=[1.5994739858411084;6.1439052752998089]
  "IW{1,1}(14,:)'" : Constant  Value=[0.9410696241686205;-6.1862321704664334]
  "IW{1,1}(15,:)'" : Constant  Value=[0.48394092777361675;-6.2371231544776862]
  "IW{1,1}(16,:)'" : Constant  Value=[-5.3679839513178003;-3.2693512437524213]
  "IW{1,1}(17,:)'" : Constant  Value=[5.2006851088601982;3.4837063697083375]
  "IW{1,1}(18,:)'" : Constant  Value=[-6.2242067762949977;0.17479614241265526]
  "IW{1,1}(19,:)'" : Constant  Value=[-6.2341058754311183;-0.052970713133795241]
  "IW{1,1}(2,:)'" : Constant  Value=[-4.3121428949445368;4.490363795128042]
  "IW{1,1}(20,:)'" : Constant  Value=[5.1724895029440798;3.526999935686876]
  "IW{1,1}(3,:)'" : Constant  Value=[-4.309773494676973;-4.5418620279150348]
  "IW{1,1}(4,:)'" : Constant  Value=[1.8463269150370314;-5.9982322915400763]
  "IW{1,1}(5,:)'" : Constant  Value=[4.8313999028477417;-3.9602203277389312]
  "IW{1,1}(6,:)'" : Constant  Value=[-6.1564153431478079;1.0600482504185951]
  "IW{1,1}(7,:)'" : Constant  Value=[-0.58147426571478278;-6.2341872708453927]
  "IW{1,1}(8,:)'" : Constant  Value=[-4.6669377909102447;-4.1787401929049155]
  "IW{1,1}(9,:)'" : Constant  Value=[4.6524200944326228;4.255796580851877]
  Mux : Mux  Inputs=20
  dotprod{1..20} (20 alike) : neural/Weight Functions/dotprod
  "iz{1,1}" : Outport
  wires:
  "IW{1,1}(1,:)'"/1 -> dotprod1/1
  "pd{1,1}"/1 -> dotprod1/2, dotprod2/2, dotprod3/2, dotprod4/2, dotprod5/2, dotprod6/2, dotprod7/2, dotprod8/2, dotprod9/2, dotprod10/2, dotprod11/2, dotprod12/2, dotprod13/2, dotprod14/2, dotprod15/2, dotprod16/2, dotprod17/2, dotprod18/2, dotprod19/2, dotprod20/2
  dotprod1/1 -> Mux/1
  "IW{1,1}(2,:)'"/1 -> dotprod2/1
  dotprod2/1 -> Mux/2
  "IW{1,1}(3,:)'"/1 -> dotprod3/1
  dotprod3/1 -> Mux/3
  "IW{1,1}(4,:)'"/1 -> dotprod4/1
  dotprod4/1 -> Mux/4
  "IW{1,1}(5,:)'"/1 -> dotprod5/1
  dotprod5/1 -> Mux/5
  "IW{1,1}(6,:)'"/1 -> dotprod6/1
  dotprod6/1 -> Mux/6
  "IW{1,1}(7,:)'"/1 -> dotprod7/1
  dotprod7/1 -> Mux/7
  "IW{1,1}(8,:)'"/1 -> dotprod8/1
  dotprod8/1 -> Mux/8
  "IW{1,1}(9,:)'"/1 -> dotprod9/1
  dotprod9/1 -> Mux/9
  "IW{1,1}(10,:)'"/1 -> dotprod10/1
  dotprod10/1 -> Mux/10
  "IW{1,1}(11,:)'"/1 -> dotprod11/1
  dotprod11/1 -> Mux/11
  "IW{1,1}(12,:)'"/1 -> dotprod12/1
  dotprod12/1 -> Mux/12
  "IW{1,1}(13,:)'"/1 -> dotprod13/1
  dotprod13/1 -> Mux/13
  "IW{1,1}(14,:)'"/1 -> dotprod14/1
  dotprod14/1 -> Mux/14
  "IW{1,1}(15,:)'"/1 -> dotprod15/1
  dotprod15/1 -> Mux/15
  "IW{1,1}(16,:)'"/1 -> dotprod16/1
  dotprod16/1 -> Mux/16
  "IW{1,1}(17,:)'"/1 -> dotprod17/1
  dotprod17/1 -> Mux/17
  "IW{1,1}(18,:)'"/1 -> dotprod18/1
  dotprod18/1 -> Mux/18
  "IW{1,1}(19,:)'"/1 -> dotprod19/1
  dotprod19/1 -> Mux/19
  "IW{1,1}(20,:)'"/1 -> dotprod20/1
  dotprod20/1 -> Mux/20
  Mux/1 -> "iz{1,1}"/1

== system hyd_hyb_2_int_cont_Final/controller1/optimized controller/SOC under 0.5/col_e_f/net_col_e_f_4_5/Layer 2/Delays 1 ==
  "p{2}" : Inport  PortDimensions=20
  mux : Mux  Inputs=1
  "pd{2,1}" : Outport
  wires:
  "p{2}"/1 -> mux/1
  mux/1 -> "pd{2,1}"/1
